simulink model "APB_Model0_v03_Test"  (R2020b)
settings: Solver=ode45  StartTime=0.0  StopTime=inf  RelTol=1e-3
undefined symbols (not defined in the file or in its folder): calb_Driver_acce, calb_Driver_bttn, calb_Driver_EmrBrk, calb_Driver_Prss, G_Fclamp, G_Kmot, G_Rmot, G_Stroke, G_SwOmega, GEN3, PbcDataStorageRequest_t
libraries: etargetslib x26, Lib_Op_Hndl x4, simulink x2, PbcOut_Checksum x2
(part 2 of 5)

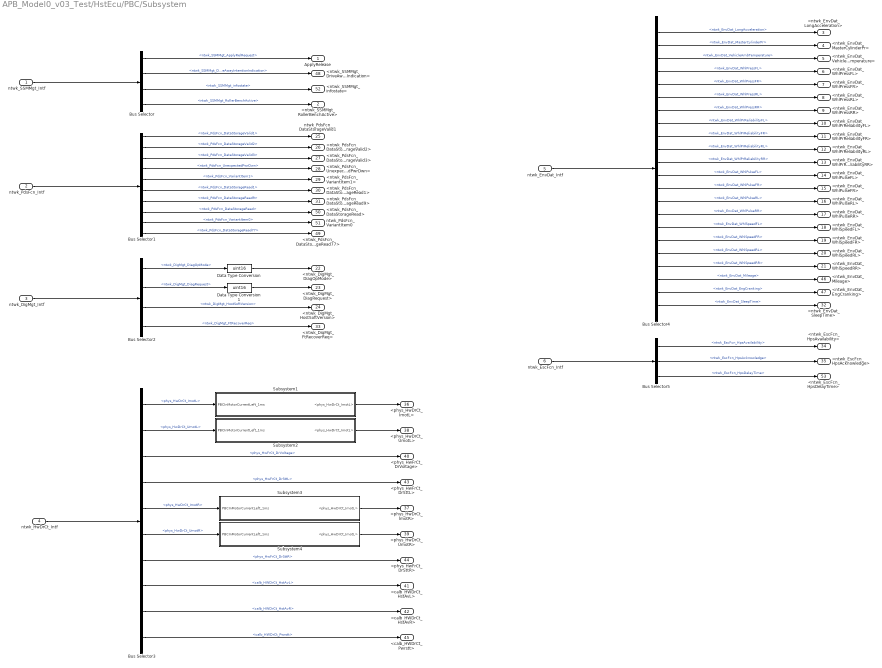
== system APB_Model0_v03_Test/HstEcu/PBC/Subsystem ==
  ntwk_SSMMgt_Intf : Inport
  ntwk_PdsFcn_Intf : Inport  Port=2
  ntwk_DigMgt_Intf : Inport  Port=3
  ntwk_HwDrCt_Intf : Inport  Port=4
  ntwk_EnvDat_Intf : Inport  Port=5
  ntwk_EscFcn_Intf : Inport  Port=6
  Bus Selector : BusSelector  OutputSignals=ntwk_SSMMgt_ApplyRelRequest,ntwk_SSMMgt_DriveAwayIntentionIndication,ntwk_SSMMgt_infostate,ntwk_SSMMgt_RollerBenchActive
  Bus Selector1 : BusSelector  OutputSignals=ntwk_PdsFcn_DataStorageValid1,ntwk_PdsFcn_DataStorageValid2,ntwk_PdsFcn_DataStorageValid3,ntwk_PdsFcn_UnexpectedPwrDwn,ntwk_PdsFcn_VariantItem1,ntwk_PdsFcn_DataStorageRead1,ntwk_PdsFcn_DataStorageRead9,ntwk_PdsFcn_DataStorageRead,ntwk_PdsFcn_VariantItem0,ntwk_PdsFcn_DataStorageRead77
  Bus Selector2 : BusSelector  OutputSignals=ntwk_DigMgt_DiagOpMode,ntwk_DigMgt_DiagRequest,ntwk_DigMgt_HostSoftVersion,ntwk_DigMgt_FtRecoverReq
  Bus Selector3 : BusSelector  OutputSignals=phys_HwDrCt_ImotL,phys_HwDrCt_UmotL,phys_HwFrCt_DrVoltage,phys_HwFrCt_DrSttL,phys_HwDrCt_ImotR,phys_HwDrCt_UmotR,phys_HwFrCt_DrSttR,calb_HWDrCt_HstAvL,calb_HWDrCt_HstAvR,calb_HWDrCt_Pwrstt
  Bus Selector4 : BusSelector  OutputSignals=ntwk_EnvDat_LongAcceleration,ntwk_EnvDat_MasterCylinderPr,ntwk_EnvDat_VehicleAmbTemperature,ntwk_EnvDat_WhlPressFL,ntwk_EnvDat_WhlPressFR,ntwk_EnvDat_WhlPressRL,ntwk_EnvDat_WhlPressRR,ntwk_EnvDat_WhlPrReliabilityFL,ntwk_EnvDat_WhlPrReliabilityFR,ntwk_EnvDat_WhlPrReliabilityRL,ntwk_EnvDat_WhlPrReliabilityRR,ntwk_EnvDat_WhlPulseFL,ntwk_EnvDat_WhlPulseFR,ntwk_EnvDat_WhlPulseRL,ntwk_EnvDat_WhlPulseRR,ntwk_EnvDat_WhlSpeedFL,ntwk_EnvDat_WhlSpeedFR,ntwk_EnvDat_WhlSpeedRL,ntwk_EnvDat_WhlSpeedRR,ntwk_EnvDat_Mileage,ntwk_EnvDat_EngCranking,ntwk_EnvDat_SleepTime
  Bus Selector5 : BusSelector  OutputSignals=ntwk_EscFcn_HpsAvailability,ntwk_EscFcn_HpsAcknowledge,ntwk_EscFcn_HpsDelayTime
  Data Type Conversion : DataTypeConversion  OutDataTypeStr=uint16
  Data Type Conversion1 : DataTypeConversion  OutDataTypeStr=uint16
  Subsystem1 : Subsystem
  Subsystem2 : Subsystem
  Subsystem3 : Subsystem
  Subsystem4 : Subsystem
  ApplyRelease : Outport
  <ntwk_SSMMgt_RollerBenchActive> : Outport  Port=2
  <ntwk_EnvDat_LongAcceleration> : Outport  Port=3
  <ntwk_EnvDat_MasterCylinderPr> : Outport  Port=4
  <ntwk_EnvDat_VehicleAmbTemperature> : Outport  Port=5
  <ntwk_EnvDat_WhlPressFL> : Outport  Port=6
  <ntwk_EnvDat_WhlPressFR> : Outport  Port=7
  <ntwk_EnvDat_WhlPressRL> : Outport  Port=8
  <ntwk_EnvDat_WhlPressRR> : Outport  Port=9
  <ntwk_EnvDat_WhlPrReliabilityFL> : Outport  Port=10
  <ntwk_EnvDat_WhlPrReliabilityFR> : Outport  Port=11
  <ntwk_EnvDat_WhlPrReliabilityRL> : Outport  Port=12
  <ntwk_EnvDat_WhlPrReliabilityRR> : Outport  Port=13
  <ntwk_EnvDat_WhlPulseFL> : Outport  Port=14
  <ntwk_EnvDat_WhlPulseFR> : Outport  Port=15
  <ntwk_EnvDat_WhlPulseRL> : Outport  Port=16
  <ntwk_EnvDat_WhlPulseRR> : Outport  Port=17
  <ntwk_EnvDat_WhlSpeedFL> : Outport  Port=18
  <ntwk_EnvDat_WhlSpeedFR> : Outport  Port=19
  <ntwk_EnvDat_WhlSpeedRL> : Outport  Port=20
  <ntwk_EnvDat_WhlSpeedRR> : Outport  Port=21
  <ntwk_DigMgt_DiagOpMode> : Outport  Port=22
  <ntwk_DigMgt_DiagRequest> : Outport  Port=23
  <ntwk_DigMgt_HostSoftVersion> : Outport  Port=24
  ntwk_PdsFcn_DataStorageValid1 : Outport  Port=25
  <ntwk_PdsFcn_DataStorageValid2> : Outport  Port=26
  <ntwk_PdsFcn_DataStorageValid3> : Outport  Port=27
  <ntwk_PdsFcn_UnexpectedPwrDwn> : Outport  Port=28
  <ntwk_PdsFcn_VariantItem1> : Outport  Port=29
  <ntwk_PdsFcn_DataStorageRead1> : Outport  Port=30
  <ntwk_PdsFcn_DataStorageRead9> : Outport  Port=31
  <ntwk_EnvDat_SleepTime> : Outport  Port=32
  <ntwk_DigMgt_FtRecoverReq> : Outport  Port=33
  <ntwk_EscFcn_HpsAvailability> : Outport  Port=34
  <ntwk_EscFcn_HpsAcknowledge> : Outport  Port=35
  <phys_HwDrCt_ImotL> : Outport  Port=36
  <phys_HwDrCt_ImotR> : Outport  Port=37
  <phys_HwDrCt_UmotL> : Outport  Port=38
  <phys_HwDrCt_UmotR> : Outport  Port=39
  <phys_HwFrCt_DrVoltage> : Outport  Port=40
  <calb_HWDrCt_HstAvL> : Outport  Port=41
  <calb_HWDrCt_HstAvR> : Outport  Port=42
  <phys_HwFrCt_DrSttL> : Outport  Port=43
  <phys_HwFrCt_DrSttR> : Outport  Port=44
  <calb_HWDrCt_Pwrstt> : Outport  Port=45
  <ntwk_EnvDat_Mileage> : Outport  Port=46
  <ntwk_EnvDat_EngCranking> : Outport  Port=47
  <ntwk_SSMMgt_DriveAwayIntentionIndication> : Outport  Port=48
  <ntwk_PdsFcn_DataStorageRead77> : Outport  Port=49
  <ntwk_PdsFcn_DataStorageRead> : Outport  Port=50
  ntwk_PdsFcn_VariantItem0 : Outport  Port=51
  <ntwk_SSMMgt_infostate> : Outport  Port=52
  <ntwk_EscFcn_HpsDelayTime> : Outport  Port=53
  wires:
  ntwk_SSMMgt_Intf/1 -> Bus Selector/1
  Bus Selector/1 -> ApplyRelease/1  "<ntwk_SSMMgt_ApplyRelRequest>"
  Bus Selector/4 -> <ntwk_SSMMgt_RollerBenchActive>/1  "<ntwk_SSMMgt_RollerBenchActive>"
  Bus Selector/3 -> <ntwk_SSMMgt_infostate>/1  "<ntwk_SSMMgt_infostate>"
  Bus Selector/2 -> <ntwk_SSMMgt_DriveAwayIntentionIndication>/1  "<ntwk_SSMMgt_DriveAwayIntentionIndication>"
  ntwk_PdsFcn_Intf/1 -> Bus Selector1/1
  Bus Selector1/1 -> ntwk_PdsFcn_DataStorageValid1/1  "<ntwk_PdsFcn_DataStorageValid1>"
  Bus Selector1/2 -> <ntwk_PdsFcn_DataStorageValid2>/1  "<ntwk_PdsFcn_DataStorageValid2>"
  Bus Selector1/3 -> <ntwk_PdsFcn_DataStorageValid3>/1  "<ntwk_PdsFcn_DataStorageValid3>"
  Bus Selector1/4 -> <ntwk_PdsFcn_UnexpectedPwrDwn>/1  "<ntwk_PdsFcn_UnexpectedPwrDwn>"
  Bus Selector1/5 -> <ntwk_PdsFcn_VariantItem1>/1  "<ntwk_PdsFcn_VariantItem1>"
  Bus Selector1/6 -> <ntwk_PdsFcn_DataStorageRead1>/1  "<ntwk_PdsFcn_DataStorageRead1>"
  Bus Selector1/9 -> ntwk_PdsFcn_VariantItem0/1  "<ntwk_PdsFcn_VariantItem0>"
  Bus Selector1/8 -> <ntwk_PdsFcn_DataStorageRead>/1  "<ntwk_PdsFcn_DataStorageRead>"
  Bus Selector1/7 -> <ntwk_PdsFcn_DataStorageRead9>/1  "<ntwk_PdsFcn_DataStorageRead9>"
  ntwk_DigMgt_Intf/1 -> Bus Selector2/1
  ntwk_HwDrCt_Intf/1 -> Bus Selector3/1
  Bus Selector2/1 -> Data Type Conversion/1  "<ntwk_DigMgt_DiagOpMode>"
  Bus Selector2/2 -> Data Type Conversion1/1  "<ntwk_DigMgt_DiagRequest>"
  Bus Selector2/3 -> <ntwk_DigMgt_HostSoftVersion>/1  "<ntwk_DigMgt_HostSoftVersion>"
  Bus Selector3/1 -> Subsystem1/1(PBCInMotorCurrentLeft_1ms)  "<phys_HwDrCt_ImotL>"
  Bus Selector3/2 -> Subsystem2/1(PBCInMotorCurrentLeft_1ms)  "<phys_HwDrCt_UmotL>"
  Bus Selector3/3 -> <phys_HwFrCt_DrVoltage>/1  "<phys_HwFrCt_DrVoltage>"
  Bus Selector3/4 -> <phys_HwFrCt_DrSttL>/1  "<phys_HwFrCt_DrSttL>"
  Bus Selector3/5 -> Subsystem3/1(PBCInMotorCurrentLeft_1ms)  "<phys_HwDrCt_ImotR>"
  Bus Selector3/6 -> Subsystem4/1(PBCInMotorCurrentLeft_1ms)  "<phys_HwDrCt_UmotR>"
  Bus Selector3/7 -> <phys_HwFrCt_DrSttR>/1  "<phys_HwFrCt_DrSttR>"
  Bus Selector3/8 -> <calb_HWDrCt_HstAvL>/1  "<calb_HWDrCt_HstAvL>"
  Bus Selector3/9 -> <calb_HWDrCt_HstAvR>/1  "<calb_HWDrCt_HstAvR>"
  Bus Selector3/10 -> <calb_HWDrCt_Pwrstt>/1  "<calb_HWDrCt_Pwrstt>"
  ntwk_EnvDat_Intf/1 -> Bus Selector4/1
  Bus Selector4/4 -> <ntwk_EnvDat_WhlPressFL>/1  "<ntwk_EnvDat_WhlPressFL>"
  Bus Selector4/3 -> <ntwk_EnvDat_VehicleAmbTemperature>/1  "<ntwk_EnvDat_VehicleAmbTemperature>"
  Bus Selector4/5 -> <ntwk_EnvDat_WhlPressFR>/1  "<ntwk_EnvDat_WhlPressFR>"
  Bus Selector4/2 -> <ntwk_EnvDat_MasterCylinderPr>/1  "<ntwk_EnvDat_MasterCylinderPr>"
  Bus Selector4/6 -> <ntwk_EnvDat_WhlPressRL>/1  "<ntwk_EnvDat_WhlPressRL>"
  Bus Selector4/1 -> <ntwk_EnvDat_LongAcceleration>/1  "<ntwk_EnvDat_LongAcceleration>"
  Bus Selector4/7 -> <ntwk_EnvDat_WhlPressRR>/1  "<ntwk_EnvDat_WhlPressRR>"
  Bus Selector4/8 -> <ntwk_EnvDat_WhlPrReliabilityFL>/1  "<ntwk_EnvDat_WhlPrReliabilityFL>"
  Bus Selector4/9 -> <ntwk_EnvDat_WhlPrReliabilityFR>/1  "<ntwk_EnvDat_WhlPrReliabilityFR>"
  Bus Selector4/10 -> <ntwk_EnvDat_WhlPrReliabilityRL>/1  "<ntwk_EnvDat_WhlPrReliabilityRL>"
  Bus Selector4/11 -> <ntwk_EnvDat_WhlPrReliabilityRR>/1  "<ntwk_EnvDat_WhlPrReliabilityRR>"
  Bus Selector4/12 -> <ntwk_EnvDat_WhlPulseFL>/1  "<ntwk_EnvDat_WhlPulseFL>"
  Bus Selector4/13 -> <ntwk_EnvDat_WhlPulseFR>/1  "<ntwk_EnvDat_WhlPulseFR>"
  Bus Selector4/14 -> <ntwk_EnvDat_WhlPulseRL>/1  "<ntwk_EnvDat_WhlPulseRL>"
  Bus Selector4/15 -> <ntwk_EnvDat_WhlPulseRR>/1  "<ntwk_EnvDat_WhlPulseRR>"
  Bus Selector4/16 -> <ntwk_EnvDat_WhlSpeedFL>/1  "<ntwk_EnvDat_WhlSpeedFL>"
  Bus Selector4/17 -> <ntwk_EnvDat_WhlSpeedFR>/1  "<ntwk_EnvDat_WhlSpeedFR>"
  Bus Selector4/18 -> <ntwk_EnvDat_WhlSpeedRL>/1  "<ntwk_EnvDat_WhlSpeedRL>"
  Bus Selector4/19 -> <ntwk_EnvDat_WhlSpeedRR>/1  "<ntwk_EnvDat_WhlSpeedRR>"
  Bus Selector4/22 -> <ntwk_EnvDat_SleepTime>/1  "<ntwk_EnvDat_SleepTime>"
  Bus Selector4/20 -> <ntwk_EnvDat_Mileage>/1  "<ntwk_EnvDat_Mileage>"
  Bus Selector4/21 -> <ntwk_EnvDat_EngCranking>/1  "<ntwk_EnvDat_EngCranking>"
  ntwk_EscFcn_Intf/1 -> Bus Selector5/1
  Bus Selector5/1 -> <ntwk_EscFcn_HpsAvailability>/1  "<ntwk_EscFcn_HpsAvailability>"
  Bus Selector5/2 -> <ntwk_EscFcn_HpsAcknowledge>/1  "<ntwk_EscFcn_HpsAcknowledge>"
  Bus Selector5/3 -> <ntwk_EscFcn_HpsDelayTime>/1  "<ntwk_EscFcn_HpsDelayTime>"
  Bus Selector2/4 -> <ntwk_DigMgt_FtRecoverReq>/1  "<ntwk_DigMgt_FtRecoverReq>"
  Bus Selector1/10 -> <ntwk_PdsFcn_DataStorageRead77>/1  "<ntwk_PdsFcn_DataStorageRead77>"
  Subsystem1/1(<phys_HwDrCt_ImotL>) -> <phys_HwDrCt_ImotL>/1
  Subsystem2/1(<phys_HwDrCt_ImotL>) -> <phys_HwDrCt_UmotL>/1
  Subsystem3/1(<phys_HwDrCt_ImotL>) -> <phys_HwDrCt_ImotR>/1
  Subsystem4/1(<phys_HwDrCt_ImotL>) -> <phys_HwDrCt_UmotR>/1
  Data Type Conversion/1 -> <ntwk_DigMgt_DiagOpMode>/1
  Data Type Conversion1/1 -> <ntwk_DigMgt_DiagRequest>/1

== system APB_Model0_v03_Test/HstEcu/PBC/Subsystem1 ==
  PBCOutActuatorStateLeft : Inport
  PBCOutActuatorStateRight : Inport  Port=2
  In3 : Inport  Port=3
  In4 : Inport  Port=4
  In5 : Inport  Port=5
  In6 : Inport  Port=6
  In7 : Inport  Port=7
  In8 : Inport  Port=8
  In9 : Inport  Port=9
  In10 : Inport  Port=10
  In11 : Inport  Port=11
  PbcSoftwareVersion : Inport  Port=12
  In1 : Inport  Port=13
  In2 : Inport  Port=14
  In12 : Inport  Port=15
  In13 : Inport  Port=16
  In14 : Inport  Port=17
  In15 : Inport  Port=18
  In16 : Inport  Port=19
  In17 : Inport  Port=20
  In18 : Inport  Port=21
  In19 : Inport  Port=22
  Bus Creator : BusCreator  Inputs=22
  PbcEsw_Intf : Outport
  wires:
  PbcSoftwareVersion/1 -> Bus Creator/1
  PBCOutActuatorStateLeft/1 -> Bus Creator/2
  PBCOutActuatorStateRight/1 -> Bus Creator/3
  Bus Creator/1 -> PbcEsw_Intf/1  "PbcEsw_Intf"
  In3/1 -> Bus Creator/4
  In4/1 -> Bus Creator/5
  In5/1 -> Bus Creator/6
  In6/1 -> Bus Creator/7
  In7/1 -> Bus Creator/8
  In8/1 -> Bus Creator/9
  In9/1 -> Bus Creator/10
  In10/1 -> Bus Creator/11
  In11/1 -> Bus Creator/12
  In1/1 -> Bus Creator/13
  In2/1 -> Bus Creator/14
  In13/1 -> Bus Creator/16
  In14/1 -> Bus Creator/17
  In15/1 -> Bus Creator/18
  In16/1 -> Bus Creator/19
  In17/1 -> Bus Creator/20
  In18/1 -> Bus Creator/21
  In19/1 -> Bus Creator/22
  In12/1 -> Bus Creator/15

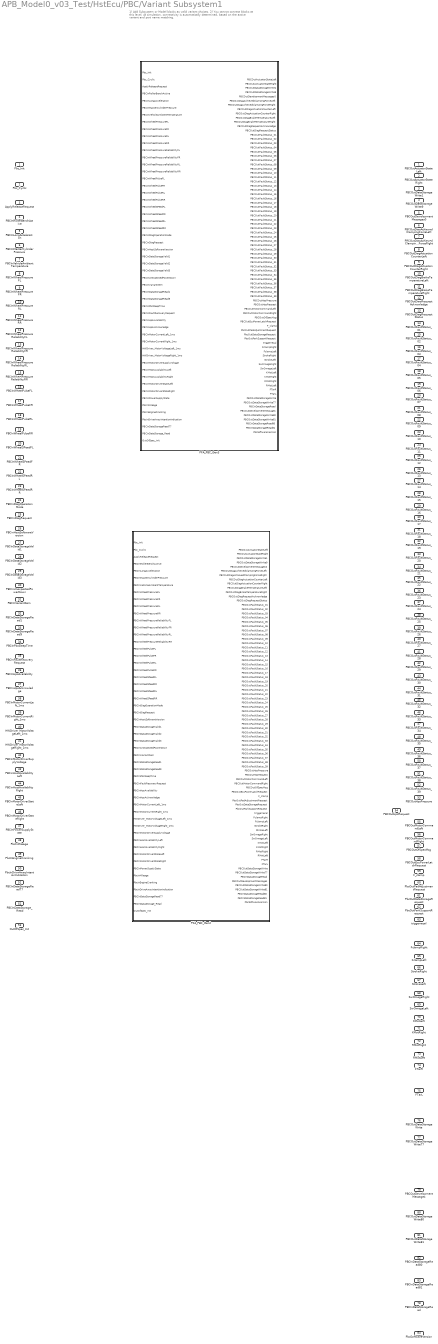
== system APB_Model0_v03_Test/HstEcu/PBC/Variant Subsystem1 ==
  note: 1) Add Subsystem or Model blocks as valid variant choices.
      | 2) You cannot connect blocks at this level. At simulation, connectivity is automatically
      | determined, based on the active variant and port name matching.
  Pbc_Init : Inport
      settings: AttributesFormatString=|
      | Type : %<OutDataTypeStr>
      | Unit : %<Unit>
  Pbc_Cyclic : Inport  Port=2
      settings: AttributesFormatString=|
      | Type : %<OutDataTypeStr>
      | Unit : %<Unit>
  ApplyReleaseRequest : Inport  Port=3
      settings: AttributesFormatString=|
      | Type : %<OutDataTypeStr>
      | Unit : %<Unit>
  PBCInRollerBenchActive : Inport  Port=4
      settings: AttributesFormatString=|
      | Type : %<OutDataTypeStr>
      | Unit : %<Unit>
  PBCInLongAcceleration : Inport  Port=5
      settings: AttributesFormatString=|
      | Type : %<OutDataTypeStr>
      | Unit : %<Unit>
  PBCInMasterCylinderPressure : Inport  Port=6
      settings: AttributesFormatString=|
      | Type : %<OutDataTypeStr>
      | Unit : %<Unit>
  PBCInVehicleAmbientTemperature : Inport  Port=7
      settings: AttributesFormatString=|
      | Type : %<OutDataTypeStr>
      | Unit : %<Unit>
  PBCInWheelPressureFL : Inport  Port=8
      settings: AttributesFormatString=|
      | Type : %<OutDataTypeStr>
      | Unit : %<Unit>
  PBCInWheelPressureFR : Inport  Port=9
      settings: AttributesFormatString=|
      | Type : %<OutDataTypeStr>
      | Unit : %<Unit>
  PBCInWheelPressureRL : Inport  Port=10
      settings: AttributesFormatString=|
      | Type : %<OutDataTypeStr>
      | Unit : %<Unit>
  PBCInWheelPressureRR : Inport  Port=11
      settings: AttributesFormatString=|
      | Type : %<OutDataTypeStr>
      | Unit : %<Unit>
  PBCInWheelPressureReliabilityFL : Inport  Port=12
      settings: AttributesFormatString=|
      | Type : %<OutDataTypeStr>
      | Unit : %<Unit>
  PBCInWheelPressureReliabilityFR : Inport  Port=13
      settings: AttributesFormatString=|
      | Type : %<OutDataTypeStr>
      | Unit : %<Unit>
  PBCInWheelPressureReliabilityRL : Inport  Port=14
      settings: AttributesFormatString=|
      | Type : %<OutDataTypeStr>
      | Unit : %<Unit>
  PBCInWheelPressureReliabilityRR : Inport  Port=15
      settings: AttributesFormatString=|
      | Type : %<OutDataTypeStr>
      | Unit : %<Unit>
  PBCInWheelPulseFL : Inport  Port=16
      settings: AttributesFormatString=|
      | Type : %<OutDataTypeStr>
      | Unit : %<Unit>
  PBCInWheelPulseFR : Inport  Port=17
      settings: AttributesFormatString=|
      | Type : %<OutDataTypeStr>
      | Unit : %<Unit>
  PBCInWheelPulseRL : Inport  Port=18
      settings: AttributesFormatString=|
      | Type : %<OutDataTypeStr>
      | Unit : %<Unit>
  PBCInWheelPulseRR : Inport  Port=19
      settings: AttributesFormatString=|
      | Type : %<OutDataTypeStr>
      | Unit : %<Unit>
  PBCInWheelSPeedFL : Inport  Port=20
      settings: AttributesFormatString=|
      | Type : %<OutDataTypeStr>
      | Unit : %<Unit>
  PBCInWheelSPeedFR : Inport  Port=21
      settings: AttributesFormatString=|
      | Type : %<OutDataTypeStr>
      | Unit : %<Unit>
  PBCInWheelSPeedRL : Inport  Port=22
      settings: AttributesFormatString=|
      | Type : %<OutDataTypeStr>
      | Unit : %<Unit>
  PBCInWheelSPeedRR : Inport  Port=23
      settings: AttributesFormatString=|
      | Type : %<OutDataTypeStr>
      | Unit : %<Unit>
  PBCInDiagOperationMode : Inport  Port=24
      settings: AttributesFormatString=|
      | Type : %<OutDataTypeStr>
      | Unit : %<Unit>
  PBCInDiagRequest : Inport  Port=25
      settings: AttributesFormatString=|
      | Type : %<OutDataTypeStr>
      | Unit : %<Unit>
  PBCinHostSoftwareVersion : Inport  Port=26
      settings: AttributesFormatString=|
      | Type : %<OutDataTypeStr>
      | Unit : %<Unit>
  PBCInDataStorageValid1 : Inport  Port=27
      settings: AttributesFormatString=|
      | Type : %<OutDataTypeStr>
      | Unit : %<Unit>
  PBCInDataStorageValid2 : Inport  Port=28
      settings: AttributesFormatString=|
      | Type : %<OutDataTypeStr>
      | Unit : %<Unit>
  PBCInDataStorageValid3 : Inport  Port=29
      settings: AttributesFormatString=|
      | Type : %<OutDataTypeStr>
      | Unit : %<Unit>
  PBCInUnexpectedPowerDown : Inport  Port=30
      settings: AttributesFormatString=|
      | Type : %<OutDataTypeStr>
      | Unit : %<Unit>
  PBCInVariantItem : Inport  Port=31
      settings: AttributesFormatString=|
      | Type : %<OutDataTypeStr>
      | Unit : %<Unit>
  PBCInDataStorageRead1 : Inport  Port=32
      settings: AttributesFormatString=|
      | Type : %<OutDataTypeStr>
      | Unit : %<Unit>
  PBCInDataStorageRead9 : Inport  Port=33
      settings: AttributesFormatString=|
      | Type : %<OutDataTypeStr>
      | Unit : %<Unit>
  PBCInPbcSleepTime : Inport  Port=34
      settings: AttributesFormatString=|
      | Type : %<OutDataTypeStr>
      | Unit : %<Unit>
  PBCInFaultRecoveryRequest : Inport  Port=35
      settings: AttributesFormatString=|
      | Type : %<OutDataTypeStr>
      | Unit : %<Unit>
  PBCInHpsAvailability : Inport  Port=36
      settings: AttributesFormatString=|
      | Type : %<OutDataTypeStr>
      | Unit : %<Unit>
  PBCInHpsAcknowledge : Inport  Port=37
      settings: AttributesFormatString=|
      | Type : %<OutDataTypeStr>
      | Unit : %<Unit>
  PBCInMotorCurrentLeft_1ms : Inport  Port=38
      settings: AttributesFormatString=|
      | Type : %<OutDataTypeStr>
      | Unit : %<Unit>
  PBCInMotorCurrentRight_1ms : Inport  Port=39
      settings: AttributesFormatString=|
      | Type : %<OutDataTypeStr>
      | Unit : %<Unit>
  HWDriver_MotorVoltageLeft_1ms : Inport  Port=40
      settings: AttributesFormatString=|
      | Type : %<OutDataTypeStr>
      | Unit : %<Unit>
  HWDriver_MotorVoltageRight_1ms : Inport  Port=41
      settings: AttributesFormatString=|
      | Type : %<OutDataTypeStr>
      | Unit : %<Unit>
  PBCInMotorDriverSupplyVoltage : Inport  Port=42
      settings: AttributesFormatString=|
      | Type : %<OutDataTypeStr>
      | Unit : %<Unit>
  PBCinHostAvailabilityLeft : Inport  Port=43
      settings: AttributesFormatString=|
      | Type : %<OutDataTypeStr>
      | Unit : %<Unit>
  PBCinHostAvailabilityRight : Inport  Port=44
      settings: AttributesFormatString=|
      | Type : %<OutDataTypeStr>
      | Unit : %<Unit>
  PBCInMotorDriverStateLeft : Inport  Port=45
      settings: AttributesFormatString=|
      | Type : %<OutDataTypeStr>
      | Unit : %<Unit>
  PBCInMotorDriverStateRight : Inport  Port=46
      settings: AttributesFormatString=|
      | Type : %<OutDataTypeStr>
      | Unit : %<Unit>
  PBCInPowerSupplyState : Inport  Port=47
      settings: AttributesFormatString=|
      | Type : %<OutDataTypeStr>
      | Unit : %<Unit>
  PbcInMileage : Inport  Port=48
      settings: AttributesFormatString=|
      | Type : %<OutDataTypeStr>
      | Unit : %<Unit>
  PbcInEngineCranking : Inport  Port=49
      settings: AttributesFormatString=|
      | Type : %<OutDataTypeStr>
      | Unit : %<Unit>
  PbcInDriveAwayIntentionIndication : Inport  Port=50
      settings: AttributesFormatString=|
      | Type : %<OutDataTypeStr>
      | Unit : %<Unit>
  PBCInDataStorageRead77 : Inport  Port=51
      settings: AttributesFormatString=|
      | Type : %<OutDataTypeStr>
      | Unit : %<Unit>
  PBCInDataStorage_Read : Inport  Port=52
      settings: AttributesFormatString=|
      | Type : %<OutDataTypeStr>
      | Unit : %<Unit>
  OutOfSpec_Init : Inport  Port=53
  PFA_PBC_Gen2 : Subsystem  VariantControl=(default)
  PFA_PBC_Gen3 : Subsystem  VariantControl=GEN3 == 1
  PBCOutActuatorStateLeft : Outport  VectorParamsAs1DForOutWhenUnconnected=off
      settings: AttributesFormatString=|
      | Type : %<OutDataTypeStr>\nInit :%<InitialOutput>
      | Unit : %<Unit>
  PBCOutActuatorStateRight : Outport  Port=2  VectorParamsAs1DForOutWhenUnconnected=off
      settings: AttributesFormatString=|
      | Type : %<OutDataTypeStr>\nInit :%<InitialOutput>
      | Unit : %<Unit>
  PBCOutDataStorageWrite1 : Outport  Port=3  VectorParamsAs1DForOutWhenUnconnected=off
      settings: AttributesFormatString=|
      | Type : %<OutDataTypeStr>\nInit :%<InitialOutput>
      | Unit : %<Unit>
  PBCOutDataStorageWrite9 : Outport  Port=4  VectorParamsAs1DForOutWhenUnconnected=off
      settings: AttributesFormatString=|
      | Type : %<OutDataTypeStr>\nInit :%<InitialOutput>
      | Unit : %<Unit>
  PBCOutDevelopmentMessages0 : Outport  Port=5  VectorParamsAs1DForOutWhenUnconnected=off
      settings: AttributesFormatString=|
      | Type : %<OutDataTypeStr>\nInit :%<InitialOutput>
      | Unit : %<Unit>
  PBCOutDiagAchievedClampingForceLeft : Outport  Port=6  VectorParamsAs1DForOutWhenUnconnected=off
      settings: AttributesFormatString=|
      | Type : %<OutDataTypeStr>\nInit :%<InitialOutput>
      | Unit : %<Unit>
  PBCOutDiagAchievedClampingForceRight : Outport  Port=7  VectorParamsAs1DForOutWhenUnconnected=off
      settings: AttributesFormatString=|
      | Type : %<OutDataTypeStr>\nInit :%<InitialOutput>
      | Unit : %<Unit>
  PBCOutDiagActuationCounterLeft : Outport  Port=8  VectorParamsAs1DForOutWhenUnconnected=off
      settings: AttributesFormatString=|
      | Type : %<OutDataTypeStr>\nInit :%<InitialOutput>
      | Unit : %<Unit>
  PBCOutDiagActuationCounterRight : Outport  Port=9  VectorParamsAs1DForOutWhenUnconnected=off
      settings: AttributesFormatString=|
      | Type : %<OutDataTypeStr>\nInit :%<InitialOutput>
      | Unit : %<Unit>
  PBCOutDiagBrakeTemperatureLeft : Outport  Port=10  VectorParamsAs1DForOutWhenUnconnected=off
      settings: AttributesFormatString=|
      | Type : %<OutDataTypeStr>\nInit :%<InitialOutput>
      | Unit : %<Unit>
  PBCOutDiagBrakeTemperatureRight : Outport  Port=11  VectorParamsAs1DForOutWhenUnconnected=off
      settings: AttributesFormatString=|
      | Type : %<OutDataTypeStr>\nInit :%<InitialOutput>
      | Unit : %<Unit>
  PBCOutDiagRequestAcknowledge : Outport  Port=12  VectorParamsAs1DForOutWhenUnconnected=off
      settings: AttributesFormatString=|
      | Type : %<OutDataTypeStr>\nInit :%<InitialOutput>
      | Unit : %<Unit>
  PBCOutDiagRequestStatus : Outport  Port=13  VectorParamsAs1DForOutWhenUnconnected=off
      settings: AttributesFormatString=|
      | Type : %<OutDataTypeStr>\nInit :%<InitialOutput>
      | Unit : %<Unit>
  PBCOutFaultStatus_01 : Outport  Port=14  VectorParamsAs1DForOutWhenUnconnected=off
      settings: AttributesFormatString=|
      | Type : %<OutDataTypeStr>\nInit :%<InitialOutput>
      | Unit : %<Unit>
  PBCOutFaultStatus_02 : Outport  Port=15  VectorParamsAs1DForOutWhenUnconnected=off
      settings: AttributesFormatString=|
      | Type : %<OutDataTypeStr>\nInit :%<InitialOutput>
      | Unit : %<Unit>
  PBCOutFaultStatus_03 : Outport  Port=16  VectorParamsAs1DForOutWhenUnconnected=off
      settings: AttributesFormatString=|
      | Type : %<OutDataTypeStr>\nInit :%<InitialOutput>
      | Unit : %<Unit>
  PBCOutFaultStatus_04 : Outport  Port=17  VectorParamsAs1DForOutWhenUnconnected=off
      settings: AttributesFormatString=|
      | Type : %<OutDataTypeStr>\nInit :%<InitialOutput>
      | Unit : %<Unit>
  PBCOutFaultStatus_05 : Outport  Port=18  VectorParamsAs1DForOutWhenUnconnected=off
      settings: AttributesFormatString=|
      | Type : %<OutDataTypeStr>\nInit :%<InitialOutput>
      | Unit : %<Unit>
  PBCOutFaultStatus_06 : Outport  Port=19  VectorParamsAs1DForOutWhenUnconnected=off
      settings: AttributesFormatString=|
      | Type : %<OutDataTypeStr>\nInit :%<InitialOutput>
      | Unit : %<Unit>
  PBCOutFaultStatus_07 : Outport  Port=20  VectorParamsAs1DForOutWhenUnconnected=off
      settings: AttributesFormatString=|
      | Type : %<OutDataTypeStr>\nInit :%<InitialOutput>
      | Unit : %<Unit>
  PBCOutFaultStatus_08 : Outport  Port=21  VectorParamsAs1DForOutWhenUnconnected=off
      settings: AttributesFormatString=|
      | Type : %<OutDataTypeStr>\nInit :%<InitialOutput>
      | Unit : %<Unit>
  PBCOutFaultStatus_09 : Outport  Port=22  VectorParamsAs1DForOutWhenUnconnected=off
      settings: AttributesFormatString=|
      | Type : %<OutDataTypeStr>\nInit :%<InitialOutput>
      | Unit : %<Unit>
  PBCOutFaultStatus_10 : Outport  Port=23  VectorParamsAs1DForOutWhenUnconnected=off
      settings: AttributesFormatString=|
      | Type : %<OutDataTypeStr>\nInit :%<InitialOutput>
      | Unit : %<Unit>
  PBCOutFaultStatus_11 : Outport  Port=24  VectorParamsAs1DForOutWhenUnconnected=off
      settings: AttributesFormatString=|
      | Type : %<OutDataTypeStr>\nInit :%<InitialOutput>
      | Unit : %<Unit>
  PBCOutFaultStatus_12 : Outport  Port=25  VectorParamsAs1DForOutWhenUnconnected=off
      settings: AttributesFormatString=|
      | Type : %<OutDataTypeStr>\nInit :%<InitialOutput>
      | Unit : %<Unit>
  PBCOutFaultStatus_13 : Outport  Port=26  VectorParamsAs1DForOutWhenUnconnected=off
      settings: AttributesFormatString=|
      | Type : %<OutDataTypeStr>\nInit :%<InitialOutput>
      | Unit : %<Unit>
  PBCOutFaultStatus_14 : Outport  Port=27  VectorParamsAs1DForOutWhenUnconnected=off
      settings: AttributesFormatString=|
      | Type : %<OutDataTypeStr>\nInit :%<InitialOutput>
      | Unit : %<Unit>
  PBCOutFaultStatus_15 : Outport  Port=28  VectorParamsAs1DForOutWhenUnconnected=off
      settings: AttributesFormatString=|
      | Type : %<OutDataTypeStr>\nInit :%<InitialOutput>
      | Unit : %<Unit>
  PBCOutFaultStatus_16 : Outport  Port=29  VectorParamsAs1DForOutWhenUnconnected=off
      settings: AttributesFormatString=|
      | Type : %<OutDataTypeStr>\nInit :%<InitialOutput>
      | Unit : %<Unit>
  PBCOutFaultStatus_17 : Outport  Port=30  VectorParamsAs1DForOutWhenUnconnected=off
      settings: AttributesFormatString=|
      | Type : %<OutDataTypeStr>\nInit :%<InitialOutput>
      | Unit : %<Unit>
  PBCOutFaultStatus_18 : Outport  Port=31  VectorParamsAs1DForOutWhenUnconnected=off
      settings: AttributesFormatString=|
      | Type : %<OutDataTypeStr>\nInit :%<InitialOutput>
      | Unit : %<Unit>
  PBCOutFaultStatus_19 : Outport  Port=32  VectorParamsAs1DForOutWhenUnconnected=off
      settings: AttributesFormatString=|
      | Type : %<OutDataTypeStr>\nInit :%<InitialOutput>
      | Unit : %<Unit>
  PBCOutFaultStatus_20 : Outport  Port=33  VectorParamsAs1DForOutWhenUnconnected=off
      settings: AttributesFormatString=|
      | Type : %<OutDataTypeStr>\nInit :%<InitialOutput>
      | Unit : %<Unit>
  PBCOutFaultStatus_21 : Outport  Port=34  VectorParamsAs1DForOutWhenUnconnected=off
      settings: AttributesFormatString=|
      | Type : %<OutDataTypeStr>\nInit :%<InitialOutput>
      | Unit : %<Unit>
  PBCOutFaultStatus_22 : Outport  Port=35  VectorParamsAs1DForOutWhenUnconnected=off
      settings: AttributesFormatString=|
      | Type : %<OutDataTypeStr>\nInit :%<InitialOutput>
      | Unit : %<Unit>
  PBCOutFaultStatus_23 : Outport  Port=36  VectorParamsAs1DForOutWhenUnconnected=off
      settings: AttributesFormatString=|
      | Type : %<OutDataTypeStr>\nInit :%<InitialOutput>
      | Unit : %<Unit>
  PBCOutFaultStatus_24 : Outport  Port=37  VectorParamsAs1DForOutWhenUnconnected=off
      settings: AttributesFormatString=|
      | Type : %<OutDataTypeStr>\nInit :%<InitialOutput>
      | Unit : %<Unit>
  PBCOutFaultStatus_25 : Outport  Port=38  VectorParamsAs1DForOutWhenUnconnected=off
      settings: AttributesFormatString=|
      | Type : %<OutDataTypeStr>\nInit :%<InitialOutput>
      | Unit : %<Unit>
  PBCOutFaultStatus_26 : Outport  Port=39  VectorParamsAs1DForOutWhenUnconnected=off
      settings: AttributesFormatString=|
      | Type : %<OutDataTypeStr>\nInit :%<InitialOutput>
      | Unit : %<Unit>
  PBCOutFaultStatus_27 : Outport  Port=40  VectorParamsAs1DForOutWhenUnconnected=off
      settings: AttributesFormatString=|
      | Type : %<OutDataTypeStr>\nInit :%<InitialOutput>
      | Unit : %<Unit>
  PBCOutFaultStatus_28 : Outport  Port=41  VectorParamsAs1DForOutWhenUnconnected=off
      settings: AttributesFormatString=|
      | Type : %<OutDataTypeStr>\nInit :%<InitialOutput>
      | Unit : %<Unit>
  PBCOutFaultStatus_29 : Outport  Port=42  VectorParamsAs1DForOutWhenUnconnected=off
      settings: AttributesFormatString=|
      | Type : %<OutDataTypeStr>\nInit :%<InitialOutput>
      | Unit : %<Unit>
  PBCOutFaultStatus_30 : Outport  Port=43  VectorParamsAs1DForOutWhenUnconnected=off
      settings: AttributesFormatString=|
      | Type : %<OutDataTypeStr>\nInit :%<InitialOutput>
      | Unit : %<Unit>
  PBCOutFaultStatus_31 : Outport  Port=44  VectorParamsAs1DForOutWhenUnconnected=off
      settings: AttributesFormatString=|
      | Type : %<OutDataTypeStr>\nInit :%<InitialOutput>
      | Unit : %<Unit>
  PBCOutFaultStatus_32 : Outport  Port=45  VectorParamsAs1DForOutWhenUnconnected=off
      settings: AttributesFormatString=|
      | Type : %<OutDataTypeStr>\nInit :%<InitialOutput>
      | Unit : %<Unit>
  PBCOutFaultStatus_33 : Outport  Port=46  VectorParamsAs1DForOutWhenUnconnected=off
      settings: AttributesFormatString=|
      | Type : %<OutDataTypeStr>\nInit :%<InitialOutput>
      | Unit : %<Unit>
  PBCOutFaultStatus_34 : Outport  Port=47  VectorParamsAs1DForOutWhenUnconnected=off
      settings: AttributesFormatString=|
      | Type : %<OutDataTypeStr>\nInit :%<InitialOutput>
      | Unit : %<Unit>
  PBCOutFaultStatus_35 : Outport  Port=48  VectorParamsAs1DForOutWhenUnconnected=off
      settings: AttributesFormatString=|
      | Type : %<OutDataTypeStr>\nInit :%<InitialOutput>
      | Unit : %<Unit>
  PBCOutFaultStatus_36 : Outport  Port=49  VectorParamsAs1DForOutWhenUnconnected=off
      settings: AttributesFormatString=|
      | Type : %<OutDataTypeStr>\nInit :%<InitialOutput>
      | Unit : %<Unit>
  PBCOutFaultStatus_37 : Outport  Port=50  VectorParamsAs1DForOutWhenUnconnected=off
      settings: AttributesFormatString=|
      | Type : %<OutDataTypeStr>\nInit :%<InitialOutput>
      | Unit : %<Unit>
  PBCOutFaultStatus_38 : Outport  Port=51  VectorParamsAs1DForOutWhenUnconnected=off
      settings: AttributesFormatString=|
      | Type : %<OutDataTypeStr>\nInit :%<InitialOutput>
      | Unit : %<Unit>
  PBCOutFaultStatus_39 : Outport  Port=52  VectorParamsAs1DForOutWhenUnconnected=off
      settings: AttributesFormatString=|
      | Type : %<OutDataTypeStr>\nInit :%<InitialOutput>
      | Unit : %<Unit>
  PBCOutHpsPressure : Outport  Port=53  VectorParamsAs1DForOutWhenUnconnected=off
      settings: AttributesFormatString=|
      | Type : %<OutDataTypeStr>\nInit :%<InitialOutput>
      | Unit : %<Unit>
  PBCOutHpsRequest : Outport  Port=54  VectorParamsAs1DForOutWhenUnconnected=off
      settings: AttributesFormatString=|
      | Type : %<OutDataTypeStr>\nInit :%<InitialOutput>
      | Unit : %<Unit>
  PBCOutMotorCommandLeft : Outport  Port=55  VectorParamsAs1DForOutWhenUnconnected=off
      settings: AttributesFormatString=|
      | Type : %<OutDataTypeStr>\nInit :%<InitialOutput>
      | Unit : %<Unit>
  PBCOutMotorCommandRight : Outport  Port=56  VectorParamsAs1DForOutWhenUnconnected=off
      settings: AttributesFormatString=|
      | Type : %<OutDataTypeStr>\nInit :%<InitialOutput>
      | Unit : %<Unit>
  PBCOutOfSpecMsg : Outport  Port=57  VectorParamsAs1DForOutWhenUnconnected=off
      settings: AttributesFormatString=|
      | Type : %<OutDataTypeStr>\nInit :%<InitialOutput>
      | Unit : %<Unit>
  PBCOutEcuPowerLatchRequest : Outport  Port=58  VectorParamsAs1DForOutWhenUnconnected=off
      settings: AttributesFormatString=|
      | Type : %<OutDataTypeStr>\nInit :%<InitialOutput>
      | Unit : %<Unit>
  F_clamp : Outport  Port=59  VectorParamsAs1DForOutWhenUnconnected=off
      settings: AttributesFormatString=|
      | Type : %<OutDataTypeStr>\nInit :%<InitialOutput>
      | Unit : %<Unit>
  PbcOutPadAdjustmentRequest : Outport  Port=60  VectorParamsAs1DForOutWhenUnconnected=off
      settings: AttributesFormatString=|
      | Type : %<OutDataTypeStr>\nInit :%<InitialOutput>
      | Unit : %<Unit>
  PbcOutDataStorageRequest : Outport  Port=61  VectorParamsAs1DForOutWhenUnconnected=off
      settings: AttributesFormatString=|
      | Type : %<OutDataTypeStr>\nInit :%<InitialOutput>
      | Unit : %<Unit>
  PbcOutParkSupportRequest : Outport  Port=62  VectorParamsAs1DForOutWhenUnconnected=off
      settings: AttributesFormatString=|
      | Type : %<OutDataTypeStr>\nInit :%<InitialOutput>
      | Unit : %<Unit>
  triggerrecal : Outport  Port=63  VectorParamsAs1DForOutWhenUnconnected=off
      settings: AttributesFormatString=|
      | Type : %<OutDataTypeStr>\nInit :%<InitialOutput>
      | Unit : %<Unit>
  FclampRight : Outport  Port=64  VectorParamsAs1DForOutWhenUnconnected=off
      settings: AttributesFormatString=|
      | Type : %<OutDataTypeStr>\nInit :%<InitialOutput>
      | Unit : %<Unit>
  FclampLeft : Outport  Port=65  VectorParamsAs1DForOutWhenUnconnected=off
      settings: AttributesFormatString=|
      | Type : %<OutDataTypeStr>\nInit :%<InitialOutput>
      | Unit : %<Unit>
  StrokeRight : Outport  Port=66  VectorParamsAs1DForOutWhenUnconnected=off
      settings: AttributesFormatString=|
      | Type : %<OutDataTypeStr>\nInit :%<InitialOutput>
      | Unit : %<Unit>
  StrokeLeft : Outport  Port=67  VectorParamsAs1DForOutWhenUnconnected=off
      settings: AttributesFormatString=|
      | Type : %<OutDataTypeStr>\nInit :%<InitialOutput>
      | Unit : %<Unit>
  SwOmegaRight : Outport  Port=68  VectorParamsAs1DForOutWhenUnconnected=off
      settings: AttributesFormatString=|
      | Type : %<OutDataTypeStr>\nInit :%<InitialOutput>
      | Unit : %<Unit>
  SwOmegaLeft : Outport  Port=69  VectorParamsAs1DForOutWhenUnconnected=off
      settings: AttributesFormatString=|
      | Type : %<OutDataTypeStr>\nInit :%<InitialOutput>
      | Unit : %<Unit>
  KMotLeft : Outport  Port=70  VectorParamsAs1DForOutWhenUnconnected=off
      settings: AttributesFormatString=|
      | Type : %<OutDataTypeStr>\nInit :%<InitialOutput>
      | Unit : %<Unit>
  KMotRight : Outport  Port=71  VectorParamsAs1DForOutWhenUnconnected=off
      settings: AttributesFormatString=|
      | Type : %<OutDataTypeStr>\nInit :%<InitialOutput>
      | Unit : %<Unit>
  RMotRight : Outport  Port=72  VectorParamsAs1DForOutWhenUnconnected=off
      settings: AttributesFormatString=|
      | Type : %<OutDataTypeStr>\nInit :%<InitialOutput>
      | Unit : %<Unit>
  RMotLeft : Outport  Port=73  VectorParamsAs1DForOutWhenUnconnected=off
      settings: AttributesFormatString=|
      | Type : %<OutDataTypeStr>\nInit :%<InitialOutput>
      | Unit : %<Unit>
  FTarR : Outport  Port=74  VectorParamsAs1DForOutWhenUnconnected=off
      settings: AttributesFormatString=|
      | Type : %<OutDataTypeStr>\nInit :%<InitialOutput>
      | Unit : %<Unit>
  FTarL : Outport  Port=75  VectorParamsAs1DForOutWhenUnconnected=off
      settings: AttributesFormatString=|
      | Type : %<OutDataTypeStr>\nInit :%<InitialOutput>
      | Unit : %<Unit>
  PBCOutDataStorageWrite : Outport  Port=76  VectorParamsAs1DForOutWhenUnconnected=off
      settings: AttributesFormatString=|
      | Type : %<OutDataTypeStr>\nInit :%<InitialOutput>
      | Unit : %<Unit>
  PBCOutDataStorageWrite77 : Outport  Port=77  VectorParamsAs1DForOutWhenUnconnected=off
      settings: AttributesFormatString=|
      | Type : %<OutDataTypeStr>\nInit :%<InitialOutput>
      | Unit : %<Unit>
  PBCInDataStorageRead : Outport  Port=78  VectorParamsAs1DForOutWhenUnconnected=off
      settings: AttributesFormatString=|
      | Type : %<OutDataTypeStr>\nInit :%<InitialOutput>
      | Unit : %<Unit>
  PBCOutDevelopmentMessages : Outport  Port=79  VectorParamsAs1DForOutWhenUnconnected=off
      settings: AttributesFormatString=|
      | Type : %<OutDataTypeStr>\nInit :%<InitialOutput>
      | Unit : %<Unit>
  PBCOutDataStorageWrite80 : Outport  Port=80  VectorParamsAs1DForOutWhenUnconnected=off
      settings: AttributesFormatString=|
      | Type : %<OutDataTypeStr>\nInit :%<InitialOutput>
      | Unit : %<Unit>
  PBCOutDataStorageWrite81 : Outport  Port=81  VectorParamsAs1DForOutWhenUnconnected=off
      settings: AttributesFormatString=|
      | Type : %<OutDataTypeStr>\nInit :%<InitialOutput>
      | Unit : %<Unit>
  PBCInDataStorageRead80 : Outport  Port=82  VectorParamsAs1DForOutWhenUnconnected=off
      settings: AttributesFormatString=|
      | Type : %<OutDataTypeStr>\nInit :%<InitialOutput>
      | Unit : %<Unit>
  PBCInDataStorageRead81 : Outport  Port=83  VectorParamsAs1DForOutWhenUnconnected=off
      settings: AttributesFormatString=|
      | Type : %<OutDataTypeStr>\nInit :%<InitialOutput>
      | Unit : %<Unit>
  PbcSoftwareVersion : Outport  Port=84

== system APB_Model0_v03_Test/HstEcu/Ssys_HstEcu0_v01/Subsystem ==
  ntwk_Driver_Intf : Inport
  ntwk_VehBhv_Intf : Inport  Port=2
  ntwk_PbcEsw_Intf : Inport  Port=3
  ntwk_Instru_Intf : Inport  Port=4
  ntwk_RdEnvt_Intf : Inport  Port=5
  Bus Selector : BusSelector  OutputSignals=calb_Driver_bttn,calb_Driver_EmrBrk,calb_Driver_acce,calb_Driver_Prss
  Bus Selector1 : BusSelector  OutputSignals=PBCOutActuatorStateLeft,PBCOutActuatorStateRight,PbcOutPadAdjustmentRequest
  Bus Selector2 : BusSelector  OutputSignals=phys_RdEnvt_Slope
  Bus Selector3 : BusSelector  OutputSignals=Arriére_Intf.phys_VehBhv_RearSpeed,Front_Intf.phys_VehBhv_FrontSpeed
  Bus Selector4 : BusSelector  OutputSignals=Instru_ReqDefault
  Delay : Delay  DelayLength=1  InitialCondition=5  SampleTime=0.001
  Delay1 : Delay  DelayLength=1  InitialCondition=5  SampleTime=0.001
  Delay2 : Delay  DelayLength=1  InitialCondition=5  SampleTime=0.001
  Out2 : Outport
  ntwk_PbcEsw_ActSttL : Outport  Port=2
  ntwk_PbcEsw_ActSttR : Outport  Port=3
  ntwk_PbcEsw_PadAdjReq : Outport  Port=4
  Out1 : Outport  Port=5
  Out8 : Outport  Port=6
  Out6 : Outport  Port=7
  Out7 : Outport  Port=8
  Out4 : Outport  Port=9
  Out3 : Outport  Port=10
  Out5 : Outport  Port=11
  wires:
  ntwk_RdEnvt_Intf/1 -> Bus Selector2/1
  ntwk_PbcEsw_Intf/1 -> Bus Selector1/1
  ntwk_Driver_Intf/1 -> Bus Selector/1
  Bus Selector/1 -> Out2/1  "<calb_Driver_bttn>"
  Bus Selector/2 -> Out3/1  "<calb_Driver_EmrBrk>"
  ntwk_VehBhv_Intf/1 -> Bus Selector3/1
  Bus Selector3/1 -> Out1/1  "<phys_VehBhv_RearSpeed>"
  Bus Selector/3 -> Out4/1  "<calb_Driver_acce>"
  ntwk_Instru_Intf/1 -> Bus Selector4/1
  Bus Selector4/1 -> Out5/1  "<Instru_ReqDefault>"
  Bus Selector2/1 -> Out6/1  "<phys_RdEnvt_Slope>"
  Bus Selector/4 -> Out7/1  "<calb_Driver_Prss>"
  Bus Selector3/2 -> Out8/1  "<phys_VehBhv_FrontSpeed>"
  Bus Selector1/1 -> Delay/1  "<PBCOutActuatorStateLeft>"
  Bus Selector1/2 -> Delay1/1  "<PBCOutActuatorStateRight>"
  Bus Selector1/3 -> Delay2/1  "<PbcOutPadAdjustmentRequest>"
  Delay/1 -> ntwk_PbcEsw_ActSttL/1
  Delay1/1 -> ntwk_PbcEsw_ActSttR/1
  Delay2/1 -> ntwk_PbcEsw_PadAdjReq/1

== system APB_Model0_v03_Test/HstEcu/Ssys_HstEcu0_v01/Subsystem1 ==
  ntwk_PbcEsw_Intf : Inport
  ntwk_Instru_Intf : Inport  Port=2
  HydPrs_Intf : Inport  Port=3
  Bus Selector : BusSelector  OutputSignals=PBCOutHpsRequest,PBCOutHpsPressure
  Bus Selector1 : BusSelector  OutputSignals=Instru_HpsDelay
  Bus Selector2 : BusSelector  OutputSignals=phys_HydPrs_PressurePist
  Data Type Conversion : DataTypeConversion  OutDataTypeStr=uint16
  Data Type Conversion1 : DataTypeConversion
  Delay : Delay  DelayLength=1
  Delay1 : Delay  DelayLength=1  SampleTime=0.001
  Delay2 : Delay  DelayLength=1  SampleTime=0.001
  ntwk_PbcEsw_HpsReq : Outport
  Out2 : Outport  Port=2
  Out1 : Outport  Port=3
  ntwk_PbcEsw_HpsPressOut : Outport  Port=4
  wires:
  ntwk_Instru_Intf/1 -> Bus Selector1/1
  HydPrs_Intf/1 -> Bus Selector2/1
  Bus Selector1/1 -> Out1/1  "<Instru_HpsDelay>"
  Bus Selector2/1 -> Delay/1  "<phys_HydPrs_PressurePist>"
  Data Type Conversion/1 -> Out2/1
  Delay1/1 -> ntwk_PbcEsw_HpsReq/1
  Delay2/1 -> ntwk_PbcEsw_HpsPressOut/1
  Delay/1 -> Data Type Conversion/1
  ntwk_PbcEsw_Intf/1 -> Bus Selector/1
  Bus Selector/1 -> Delay1/1  "<PBCOutHpsRequest>"
  Bus Selector/2 -> Data Type Conversion1/1  "<PBCOutHpsPressure>"
  Data Type Conversion1/1 -> Delay2/1

== system APB_Model0_v03_Test/HstEcu/Ssys_HstEcu0_v01/Subsystem2 ==
  HydPrs_Intf : Inport
  ntwk_Instru_Intf : Inport  Port=2
  ntwk_VehBhv_Intf : Inport  Port=3
  ntwk_RdEnvt_Intf : Inport  Port=4
  ntwk_Driver_Intf : Inport  Port=5
  Bus Selector : BusSelector  OutputSignals=phys_HydPrs_PressurePist
  Bus Selector1 : BusSelector  OutputSignals=Arriére_Intf.phys_VehBhv_RearPulse,Front_Intf.phys_VehBhv_FrontSpeed,Arriére_Intf.phys_VehBhv_AmbTemp,Arriére_Intf.phys_VehBhv_RearSpeed,Front_Intf.phys_VehBhv_FrontPulse
  Bus Selector2 : BusSelector  OutputSignals=phys_RdEnvt_LgAc
  Bus Selector3 : BusSelector  OutputSignals=calb_Driver_Prss
  Bus Selector4 : BusSelector  OutputSignals=Instru_WhlPrsReliabTestSignalFL,Instru_WhlPrsReliabTestSignalFR,Instru_WhlPrsReliabTestSignalRL,Instru_WhlPrsReliabTestSignalRR,Instru_WhlSpdTestSignalRL,Instru_WhlSpdTestSignalRR,Instru_WhlSpdTestSignalFL,Instru_WhlSpdTestSignalFR,Instru_WhlPulsTestSignalFL,Instru_WhlPulsTestSignalFR,Instru_WhlPulsTestSignalRL,Instru_WhlPulsTestSignalRR,Instru_WhlPrsTestSignalRL,Instru_WhlPrsTestSignalRR,Instru_WhlPrsTestSignalFL,Instru_WhlPrsTestSignalFR
  Mux : Mux  Inputs=7
  X : Outport
  Out1 : Outport  Port=2
  Out3 : Outport  Port=3
  Out4 : Outport  Port=4
  Out5 : Outport  Port=5
  Out6 : Outport  Port=6
  Out7 : Outport  Port=7
  Out8 : Outport  Port=8
  Out9 : Outport  Port=9
  Out10 : Outport  Port=10
  Out11 : Outport  Port=11
  Out12 : Outport  Port=12
  Out13 : Outport  Port=13
  Out14 : Outport  Port=14
  Out15 : Outport  Port=15
  Out16 : Outport  Port=16
  Out17 : Outport  Port=17
  Out2 : Outport  Port=18
  wires:
  HydPrs_Intf/1 -> Bus Selector/1
  Bus Selector/1 -> Out2/1  "<phys_HydPrs_PressurePist>"
  ntwk_VehBhv_Intf/1 -> Bus Selector1/1
  ntwk_RdEnvt_Intf/1 -> Bus Selector2/1
  Bus Selector2/1 -> Mux/1  "<phys_RdEnvt_LgAc>"
  ntwk_Driver_Intf/1 -> Bus Selector3/1
  Bus Selector1/1 -> Mux/2  "<phys_VehBhv_RearPulse>"
  Bus Selector1/2 -> Mux/3  "<phys_VehBhv_FrontSpeed>"
  Bus Selector1/3 -> Mux/4  "<phys_VehBhv_AmbTemp>"
  Bus Selector1/4 -> Mux/5  "<phys_VehBhv_RearSpeed>"
  Bus Selector1/5 -> Mux/6  "<phys_VehBhv_FrontPulse>"
  Bus Selector3/1 -> Mux/7  "<calb_Driver_Prss>"
  Mux/1 -> X/1
  ntwk_Instru_Intf/1 -> Bus Selector4/1
  Bus Selector4/1 -> Out1/1  "<Instru_WhlPrsReliabTestSignalFL>"
  Bus Selector4/2 -> Out3/1  "<Instru_WhlPrsReliabTestSignalFR>"
  Bus Selector4/3 -> Out4/1  "<Instru_WhlPrsReliabTestSignalRL>"
  Bus Selector4/4 -> Out5/1  "<Instru_WhlPrsReliabTestSignalRR>"
  Bus Selector4/5 -> Out6/1  "<Instru_WhlSpdTestSignalRL>"
  Bus Selector4/6 -> Out7/1  "<Instru_WhlSpdTestSignalRR>"
  Bus Selector4/7 -> Out8/1  "<Instru_WhlSpdTestSignalFL>"
  Bus Selector4/8 -> Out9/1  "<Instru_WhlSpdTestSignalFR>"
  Bus Selector4/9 -> Out10/1  "<Instru_WhlPulsTestSignalFL>"
  Bus Selector4/10 -> Out11/1  "<Instru_WhlPulsTestSignalFR>"
  Bus Selector4/11 -> Out12/1  "<Instru_WhlPulsTestSignalRL>"
  Bus Selector4/12 -> Out13/1  "<Instru_WhlPulsTestSignalRR>"
  Bus Selector4/13 -> Out14/1  "<Instru_WhlPrsTestSignalRL>"
  Bus Selector4/14 -> Out15/1  "<Instru_WhlPrsTestSignalRR>"
  Bus Selector4/15 -> Out16/1  "<Instru_WhlPrsTestSignalFL>"
  Bus Selector4/16 -> Out17/1  "<Instru_WhlPrsTestSignalFR>"

== system APB_Model0_v03_Test/HstEcu/Ssys_HstEcu0_v01/Subsystem3 ==
  ntwk_SSMMgt_ApplyRelRequest : Inport
  ntwk_SSMMgt_DriveAwayIntentionIndication : Inport  Port=2
  ntwk_SSMMgt_infostate : Inport  Port=3
  ntwk_SSMMgt_RollerBenchActive : Inport  Port=4
  Bus Creator : BusCreator  Inputs=4
  ntwk_SSMMgt_Intf : Outport
  wires:
  ntwk_SSMMgt_RollerBenchActive/1 -> Bus Creator/4  "ntwk_SSMMgt_RollerBenchActive"
  ntwk_SSMMgt_infostate/1 -> Bus Creator/3  "ntwk_SSMMgt_infostate"
  ntwk_SSMMgt_DriveAwayIntentionIndication/1 -> Bus Creator/2  "ntwk_SSMMgt_DriveAwayIntentionIndication"
  ntwk_SSMMgt_ApplyRelRequest/1 -> Bus Creator/1  "ntwk_SSMMgt_ApplyRelRequest"
  Bus Creator/1 -> ntwk_SSMMgt_Intf/1

== system APB_Model0_v03_Test/HstEcu/Ssys_HstEcu0_v01/Subsystem4 ==
  ntwk_DigMgt_DiagOpMode : Inport
  ntwk_DigMgt_DiagRequest : Inport  Port=2
  In3 : Inport  Port=3
  In1 : Inport  Port=4
  Bus Creator : BusCreator  Inputs=4
  ntwk_DigMgt_Intf : Outport
  wires:
  Bus Creator/1 -> ntwk_DigMgt_Intf/1
  In3/1 -> Bus Creator/3
  ntwk_DigMgt_DiagRequest/1 -> Bus Creator/2  "ntwk_DigMgt_DiagRequest"
  ntwk_DigMgt_DiagOpMode/1 -> Bus Creator/1  "ntwk_DigMgt_DiagOpMode"
  In1/1 -> Bus Creator/4

== system APB_Model0_v03_Test/HstEcu/Ssys_HstEcu0_v01/Subsystem5 ==
  In1 : Inport
  In2 : Inport  Port=2
  In3 : Inport  Port=3
  In4 : Inport  Port=4
  In5 : Inport  Port=5
  In6 : Inport  Port=6
  In7 : Inport  Port=7
  In8 : Inport  Port=8
  In9 : Inport  Port=9
  In10 : Inport  Port=10
  Bus Creator : BusCreator  Inputs=10
  ntwk_PdsFcn_Intf : Outport
  wires:
  Bus Creator/1 -> ntwk_PdsFcn_Intf/1
  In9/1 -> Bus Creator/9
  In8/1 -> Bus Creator/8
  In7/1 -> Bus Creator/7
  In6/1 -> Bus Creator/6
  In5/1 -> Bus Creator/5
  In4/1 -> Bus Creator/4
  In3/1 -> Bus Creator/3
  In2/1 -> Bus Creator/2
  In1/1 -> Bus Creator/1
  In10/1 -> Bus Creator/10

== system APB_Model0_v03_Test/HstEcu/Ssys_HstEcu0_v01/Subsystem6 ==
  In1 : Inport
  In2 : Inport  Port=2
  In3 : Inport  Port=3
  In4 : Inport  Port=4
  In5 : Inport  Port=5
  In6 : Inport  Port=6
  In7 : Inport  Port=7
  In8 : Inport  Port=8
  In9 : Inport  Port=9
  In10 : Inport  Port=10
  In11 : Inport  Port=11
  In12 : Inport  Port=12
  In13 : Inport  Port=13
  In14 : Inport  Port=14
  In15 : Inport  Port=15
  In16 : Inport  Port=16
  In17 : Inport  Port=17
  In18 : Inport  Port=18
  In19 : Inport  Port=19
  In20 : Inport  Port=20
  In21 : Inport  Port=21
  In22 : Inport  Port=22
  Bus Creator : BusCreator  Inputs=22
  ntwk_EnvDat_Intf : Outport
  wires:
  Bus Creator/1 -> ntwk_EnvDat_Intf/1
  In22/1 -> Bus Creator/22
  In21/1 -> Bus Creator/21
  In20/1 -> Bus Creator/20
  In19/1 -> Bus Creator/19
  In18/1 -> Bus Creator/18
  In17/1 -> Bus Creator/17
  In16/1 -> Bus Creator/16
  In15/1 -> Bus Creator/15
  In14/1 -> Bus Creator/14
  In13/1 -> Bus Creator/13
  In12/1 -> Bus Creator/12
  In11/1 -> Bus Creator/11
  In10/1 -> Bus Creator/10
  In9/1 -> Bus Creator/9
  In8/1 -> Bus Creator/8
  In7/1 -> Bus Creator/7
  In6/1 -> Bus Creator/6
  In5/1 -> Bus Creator/5
  In4/1 -> Bus Creator/4
  In1/1 -> Bus Creator/1
  In2/1 -> Bus Creator/2
  In3/1 -> Bus Creator/3

== system APB_Model0_v03_Test/HstEcu/Ssys_HstEcu0_v01/Subsystem7 ==
  In1 : Inport
  In2 : Inport  Port=2
  In3 : Inport  Port=3
  Bus Creator : BusCreator  Inputs=3
  ntwk_EscFcn_Intf : Outport
  wires:
  Bus Creator/1 -> ntwk_EscFcn_Intf/1  "ntwk_EscFcn_Intf"
  In3/1 -> Bus Creator/3
  In1/1 -> Bus Creator/1
  In2/1 -> Bus Creator/2

== system APB_Model0_v03_Test/HstEcu/Ssys_HstEcu0_v01/Subsystem8 ==
  ntwk_Instru_Intf : Inport
  phys_ActMtrL_Intf : Inport  Port=2
  phys_ActMtrR_Intf : Inport  Port=3
  phys_PowerStageL_Intf : Inport  Port=4
  phys_PowerStageR_Intf : Inport  Port=5
  phys_PwrNet_Intf : Inport  Port=6
  Bus Selector : BusSelector  OutputSignals=Instru_DriVolTestSignal
  Bus Selector1 : BusSelector  OutputSignals=phys_ActMtr_Current
  Bus Selector2 : BusSelector  OutputSignals=phys_ActMtr_Current
  Bus Selector3 : BusSelector  OutputSignals=phys_ActHbdg_PBCVOLIn,phys_ActHbdg_PBCCurrIn,ntwk_PBCEsw_MotorDriverState
  Bus Selector4 : BusSelector  OutputSignals=phys_ActHbdg_PBCVOLIn,phys_ActHbdg_PBCCurrIn,ntwk_PBCEsw_MotorDriverState
  Bus Selector5 : BusSelector  OutputSignals=phys_PwrNet_VIn
  Out1 : Outport
  Out2 : Outport  Port=2
  Out3 : Outport  Port=3
  Out4 : Outport  Port=4
  Out5 : Outport  Port=5
  Out8 : Outport  Port=6
  Out6 : Outport  Port=7
  Out7 : Outport  Port=8
  wires:
  ntwk_Instru_Intf/1 -> Bus Selector/1
  phys_ActMtrL_Intf/1 -> Bus Selector1/1
  phys_ActMtrR_Intf/1 -> Bus Selector2/1
  phys_PowerStageL_Intf/1 -> Bus Selector3/1
  phys_PowerStageR_Intf/1 -> Bus Selector4/1
  Bus Selector/1 -> Out1/1  "<Instru_DriVolTestSignal>"
  Bus Selector3/3 -> Out6/1  "<ntwk_PBCEsw_MotorDriverState>"
  Bus Selector4/3 -> Out7/1  "<ntwk_PBCEsw_MotorDriverState>"
  phys_PwrNet_Intf/1 -> Bus Selector5/1
  Bus Selector5/1 -> Out8/1  "<phys_PwrNet_VIn>"
  Bus Selector3/1 -> Out2/1  "<phys_ActHbdg_PBCVOLIn>"
  Bus Selector4/1 -> Out3/1  "<phys_ActHbdg_PBCVOLIn>"
  Bus Selector1/1 -> ?  "<phys_ActMtr_Current>"
  Bus Selector2/1 -> ?  "<phys_ActMtr_Current>"
  Bus Selector3/2 -> Out4/1  "<phys_ActHbdg_PBCCurrIn>"
  Bus Selector4/2 -> Out5/1  "<phys_ActHbdg_PBCCurrIn>"

== system APB_Model0_v03_Test/HstEcu/Ssys_HstEcu0_v01/Subsystem9 ==
  In1 : Inport
  In2 : Inport  Port=2
  In3 : Inport  Port=3
  In4 : Inport  Port=4
  In5 : Inport  Port=5
  In6 : Inport  Port=6
  In7 : Inport  Port=7
  In8 : Inport  Port=8
  In9 : Inport  Port=9
  In10 : Inport  Port=10
  Bus Creator : BusCreator  Inputs=10
  ntwk_HwDrCt_Intf : Outport
  wires:
  In1/1 -> Bus Creator/1
  In2/1 -> Bus Creator/2
  In3/1 -> Bus Creator/3
  In4/1 -> Bus Creator/4
  In5/1 -> Bus Creator/5
  In6/1 -> Bus Creator/6
  In7/1 -> Bus Creator/7
  In8/1 -> Bus Creator/8
  In9/1 -> Bus Creator/9
  In10/1 -> Bus Creator/10
  Bus Creator/1 -> ntwk_HwDrCt_Intf/1

== system APB_Model0_v03_Test/HstEcu/PBC/Subsystem/Subsystem1 ==
  PBCInMotorCurrentLeft_1ms : Inport
  Constant : Constant  Value=GEN3
  Delay : Delay  DelayLength=1
  Subsystem : Subsystem
  Subsystem4 : Subsystem
  Switch : Switch  Criteria=u2 ~= 0
  <phys_HwDrCt_ImotL> : Outport
  wires:
  Constant/1 -> Switch/2
  Subsystem4/1(Out1) -> Switch/1
  Subsystem/1(Out1) -> Switch/3
  Switch/1 -> <phys_HwDrCt_ImotL>/1
  PBCInMotorCurrentLeft_1ms/1 -> Delay/1
  Delay/1 -> Subsystem4/1(PBCInMotorCurrentLeft_1ms), Subsystem/1(PBCInMotorCurrentLeft_1ms)

== system APB_Model0_v03_Test/HstEcu/PBC/Subsystem/Subsystem2 ==
  PBCInMotorCurrentLeft_1ms : Inport
  Constant : Constant  Value=GEN3
  Delay : Delay  DelayLength=1
  Subsystem : Subsystem
  Subsystem4 : Subsystem
  Switch : Switch  Criteria=u2 ~= 0
  <phys_HwDrCt_ImotL> : Outport
  wires:
  PBCInMotorCurrentLeft_1ms/1 -> Delay/1
  Switch/1 -> <phys_HwDrCt_ImotL>/1
  Subsystem/1(Out1) -> Switch/3
  Subsystem4/1(Out1) -> Switch/1
  Constant/1 -> Switch/2
  Delay/1 -> Subsystem/1(PBCInMotorCurrentLeft_1ms), Subsystem4/1(PBCInMotorCurrentLeft_1ms)
